simulink model "PenduloLinearidade"  (Simulink 7.2)
settings: Solver=ode45  StartTime=0.0  StopTime=100  RelTol=1e-3
settings Model: Creator=Leonardo  LastModifiedBy=52473520682
settings DebuggingCC: StrictBusMsg=ErrorLevel1

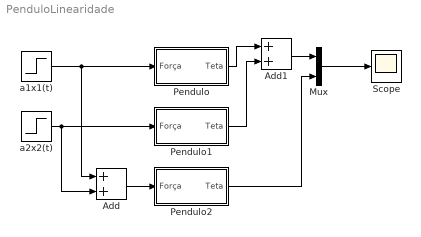
== system PenduloLinearidade ==
  Add : Sum  OutDataType=sfix(16)  OutScaling=2^-10
  Add1 : Sum  OutDataType=sfix(16)  OutScaling=2^-10
  Mux : Mux  Inputs=2
  Pendulo : Subsystem
  Pendulo1 : Subsystem
  Pendulo2 : Subsystem
  Scope : Scope
      settings: TimeRange=100  YMin=0  YMax=1
  a1x1(t) : Step  Time=0  After=0.5  SampleTime=0
  a2x2(t) : Step  Time=0  After=0.3  SampleTime=0
  wires:
  a1x1(t)/1 -> Pendulo/1(Força), Add/1
  Mux/1 -> Scope/1
  a2x2(t)/1 -> Pendulo1/1(Força), Add/2
  Add/1 -> Pendulo2/1(Força)
  Pendulo/1(Teta) -> Add1/1
  Pendulo1/1(Teta) -> Add1/2
  Add1/1 -> Mux/1
  Pendulo2/1(Teta) -> Mux/2

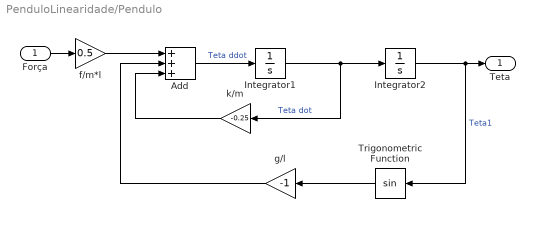
== system PenduloLinearidade/Pendulo ==
  Força : Inport
  Add : Sum  Inputs=+++
  Integrator1 : Integrator
  Integrator2 : Integrator
  Trigonometric Function : Trigonometry  Orientation=left
  f/m*l : Gain  Gain=0.5
  g/l : Gain  Orientation=left  Gain=-1
  k/m : Gain  Orientation=left  Gain=-0.25
  Teta : Outport
  wires:
  Integrator1/1 -> Integrator2/1, k/m/1  "Teta dot"
  Add/1 -> Integrator1/1  "Teta ddot"
  Integrator2/1 -> Teta/1, Trigonometric Function/1  "Teta1"
  Trigonometric Function/1 -> g/l/1
  g/l/1 -> Add/2
  k/m/1 -> Add/3
  f/m*l/1 -> Add/1
  Força/1 -> f/m*l/1

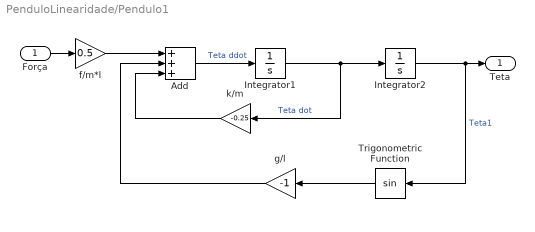
== system PenduloLinearidade/Pendulo1 ==
  Força : Inport
  Add : Sum  Inputs=+++
  Integrator1 : Integrator
  Integrator2 : Integrator
  Trigonometric Function : Trigonometry  Orientation=left
  f/m*l : Gain  Gain=0.5
  g/l : Gain  Orientation=left  Gain=-1
  k/m : Gain  Orientation=left  Gain=-0.25
  Teta : Outport
  wires:
  Integrator1/1 -> Integrator2/1, k/m/1  "Teta dot"
  Add/1 -> Integrator1/1  "Teta ddot"
  Integrator2/1 -> Teta/1, Trigonometric Function/1  "Teta1"
  Trigonometric Function/1 -> g/l/1
  g/l/1 -> Add/2
  k/m/1 -> Add/3
  f/m*l/1 -> Add/1
  Força/1 -> f/m*l/1

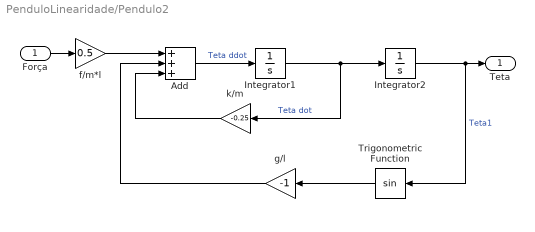
== system PenduloLinearidade/Pendulo2 ==
  Força : Inport
  Add : Sum  Inputs=+++
  Integrator1 : Integrator
  Integrator2 : Integrator
  Trigonometric Function : Trigonometry  Orientation=left
  f/m*l : Gain  Gain=0.5
  g/l : Gain  Orientation=left  Gain=-1
  k/m : Gain  Orientation=left  Gain=-0.25
  Teta : Outport
  wires:
  Integrator1/1 -> Integrator2/1, k/m/1  "Teta dot"
  Add/1 -> Integrator1/1  "Teta ddot"
  Integrator2/1 -> Teta/1, Trigonometric Function/1  "Teta1"
  Trigonometric Function/1 -> g/l/1
  g/l/1 -> Add/2
  k/m/1 -> Add/3
  f/m*l/1 -> Add/1
  Força/1 -> f/m*l/1
